simulink model "canTransceiverModel"  (R2018a)
settings: Solver=FixedStepDiscrete  StartTime=0.0  StopTime=50  RelTol=1e-3  EnableMultiTasking=on
values from neighbouring files (symbols this model uses):
  sampleTime = 0.040    (= 0.04)    [canTrasceiverConfig.m]
  sensorLocationConfig = uint8(sensorLocationConfig)    [canTrasceiverConfig.m]
undefined symbols (not defined in the file or in its folder): canChannel, CRC
libraries: simulink x81, canmsglib x27, canlib x8, commcrc2 x1
(part 1 of 5)
settings Model: FPTRunName=Active  Creator=The MathWorks, Inc.  LastModifiedBy=Giovanni
settings DataIOCC: LimitDataPoints=on  SaveFormat=Array
settings OptimizationCC: BlockReduction=off  ExpressionDepthLimit=2147483647  LifeSpan=inf
settings DebuggingCC: UnderspecifiedInitializationDetection=Classic  MergeDetectMultiDrivingBlocksExec=none  SolverPrmCheckMsg=warning  FcnCallInpInsideContextMsg=warning  StateNameClashWarn=warning  SFUnexpectedBacktrackingDiag=warning  SFNoUnconditionalDefaultTransitionDiag=warning  SFExecutionAtInitializationDiag=none
settings HardwareCC: ProdBitPerPointer=32  ProdBitPerSizeT=32  ProdBitPerPtrDiffT=32  ProdLargestAtomicFloat=None  ProdIntDivRoundTo=Undefined  ProdEndianess=Unspecified  ProdWordSize=32  ProdHWDeviceType=32-bit Generic
settings ModelReferenceCC: PropagateSignalLabelsOutOfModel=off
settings RTWCC: PostCodeGenCommand=packNGo(buildInfo)  Description=Generic Real-Time Target  RetainRTWFile=on  TLCDebug=on
settings CodeAppCC: StateflowObjectComments=on
settings GRTTargetCC: TargetLangStandard=C89/C90 (ANSI)  GeneratePreprocessorConditionals=Disable all  CombineOutputUpdateFcns=off  MatFileLogging=off  GRTInterface=on
settings ConfigComp: CovMetricSettings=dw  CovHtmlReporting=on  CovSaveCumulativeToWorkspaceVar=on  CovSaveSingleToWorkspaceVar=on  CovExternalEMLEnable=off

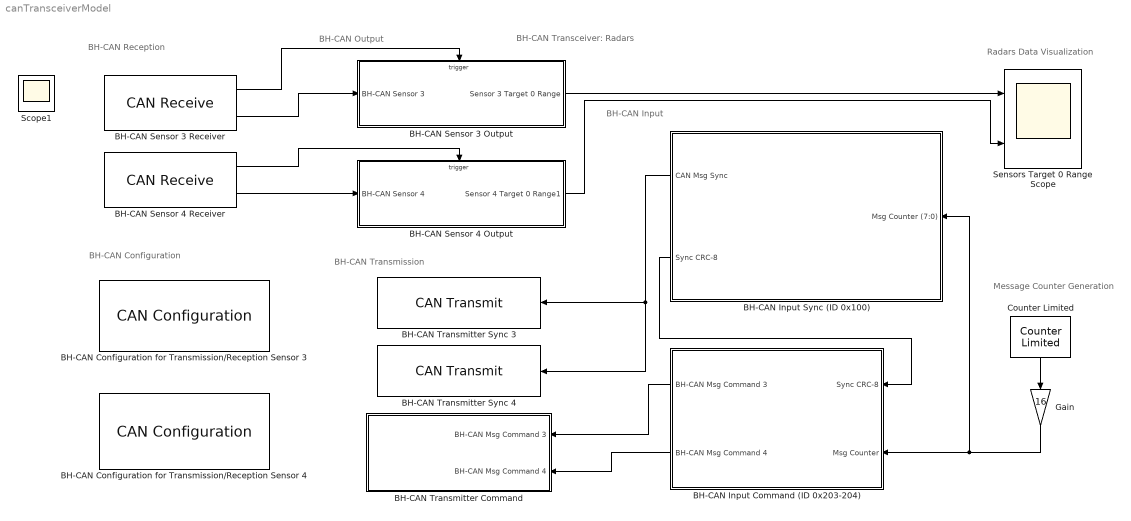
== system canTransceiverModel ==
  note: Radars Data Visualization
  note: BH-CAN Input
  note: BH-CAN Configuration
  note: BH-CAN Output
  note: BH-CAN Reception
  note: BH-CAN Transmission
  note: Message Counter
      | Generation
  note: BH-CAN Transceiver: Radars
  BH-CAN Configuration for Transmission/Reception Sensor 3 : canlib/CAN Configuration  BlockHandle=5.0001  DeviceMenu=MathWorks Virtual 1 (Channel 1)  Device=Vector VN1640A 1 (Channel 1)  ObjConstructor=canChannel('Vector','VN1640A 1',1)  BusSpeed=500000  EnableBitParameters=off  SJW=1  TSEG1=4  TSEG2=3  NSamples=1  AckMode=Normal
      settings: SourceProductName=Vehicle Network Toolbox  SourceProductBaseCode=VN
  BH-CAN Configuration for Transmission/Reception Sensor 4 : canlib/CAN Configuration  BlockHandle=6.0001  DeviceMenu=MathWorks Virtual 1 (Channel 1)  Device=Vector VN1640A 1 (Channel 2)  ObjConstructor=canChannel('Vector','VN1640A 1',2)  BusSpeed=500000  EnableBitParameters=off  SJW=1  TSEG1=4  TSEG2=3  NSamples=1  AckMode=Normal
      settings: SourceProductName=Vehicle Network Toolbox  SourceProductBaseCode=VN
  BH-CAN Input Command (ID 0x203-204) : Subsystem
  BH-CAN Input Sync (ID 0x100) : Subsystem
  BH-CAN Sensor 3 Output : Subsystem  TreatAsAtomicUnit=on
      settings: RTWSystemCode=Nonreusable function
  BH-CAN Sensor 3 Receiver : canlib/CAN Receive  BlockHandle=1800.0001  DeviceMenu=(none)  Device=Vector VN1640A 1 (Channel 1)  ObjConstructor=canChannel('Vector','VN1640A 1',1)  EnableStandardIDsFilter=off  StandardIDs=0  EnableExtendedIDsFilter=off  ExtendedIDs=0  SampleTime=sampleTime  MsgsPerTimestep=all  StdIDsCombo=Allow all  ExtIDsCombo=Allow all  InternalFilterUpdateStatus=on  BusOutput=off
      settings: SourceProductName=Vehicle Network Toolbox  SourceProductBaseCode=VN
  BH-CAN Sensor 4 Output : Subsystem  TreatAsAtomicUnit=on
      settings: RTWSystemCode=Nonreusable function
  BH-CAN Sensor 4 Receiver : canlib/CAN Receive  BlockHandle=3437.0001  DeviceMenu=MathWorks Virtual 1 (Channel 1)  Device=Vector VN1640A 1 (Channel 2)  ObjConstructor=canChannel('Vector','VN1640A 1',2)  EnableStandardIDsFilter=off  StandardIDs=0  EnableExtendedIDsFilter=off  ExtendedIDs=0  SampleTime=sampleTime  MsgsPerTimestep=all  StdIDsCombo=Allow all  ExtIDsCombo=Allow all  InternalFilterUpdateStatus=on  BusOutput=off
      settings: SourceProductName=Vehicle Network Toolbox  SourceProductBaseCode=VN
  BH-CAN Transmitter Command : Subsystem
  BH-CAN Transmitter Sync 3 : canlib/CAN Transmit  BlockHandle=3445.0001  DeviceMenu=MathWorks Virtual 1 (Channel 1)  Device=Vector VN1640A 1 (Channel 1)  ObjConstructor=canChannel('Vector','VN1640A 1',1)  EnablePeriodicTransmit=off  MessagePeriod=0.025
      settings: SourceProductName=Vehicle Network Toolbox  SourceProductBaseCode=VN
  BH-CAN Transmitter Sync 4 : canlib/CAN Transmit  BlockHandle=3446.0001  DeviceMenu=MathWorks Virtual 1 (Channel 1)  Device=Vector VN1640A 1 (Channel 2)  ObjConstructor=canChannel('Vector','VN1640A 1',2)  EnablePeriodicTransmit=off  MessagePeriod=0.025
      settings: SourceProductName=Vehicle Network Toolbox  SourceProductBaseCode=VN
  Counter Limited : simulink/Sources/Counter Limited  uplimit=15  tsamp=sampleTime
  Gain : Gain  Gain=16  OutDataTypeStr=Inherit: Same as input
  Sensors Target 0 Range Scope : Scope  NumInputPorts=2
  Scope1 : Scope
  wires:
  BH-CAN Input Sync (ID 0x100)/1(CAN Msg Sync) -> BH-CAN Transmitter Sync 3/1, BH-CAN Transmitter Sync 4/1
  Counter Limited/1 -> Gain/1
  Gain/1 -> BH-CAN Input Sync (ID 0x100)/1(Msg Counter (7:0)), BH-CAN Input Command (ID 0x203-204)/2(Msg Counter)
  BH-CAN Sensor 3 Receiver/2 -> BH-CAN Sensor 3 Output/1(BH-CAN Sensor 3)
  BH-CAN Sensor 3 Receiver/1 -> BH-CAN Sensor 3 Output/Trigger
  BH-CAN Sensor 4 Receiver/1 -> BH-CAN Sensor 4 Output/Trigger
  BH-CAN Sensor 4 Receiver/2 -> BH-CAN Sensor 4 Output/1(BH-CAN Sensor 4)
  BH-CAN Input Sync (ID 0x100)/2(Sync CRC-8) -> BH-CAN Input Command (ID 0x203-204)/1(Sync CRC-8)
  BH-CAN Input Command (ID 0x203-204)/1(BH-CAN Msg Command 3) -> BH-CAN Transmitter Command/1(BH-CAN Msg Command 3)
  BH-CAN Input Command (ID 0x203-204)/2(BH-CAN Msg Command 4) -> BH-CAN Transmitter Command/2(BH-CAN Msg Command 4)
  BH-CAN Sensor 3 Output/1(Sensor 3 Target 0 Range) -> Sensors Target 0 Range Scope/1
  BH-CAN Sensor 4 Output/1(Sensor 4 Target 0 Range1) -> Sensors Target 0 Range Scope/2

== system canTransceiverModel/BH-CAN Input Command (ID 0x203-204) ==
  Sync CRC-8 : Inport
  Msg Counter : Inport  Port=2
  BH-CAN Input Command 3 (ID 0x203) : Subsystem
  BH-CAN Input Command 4 (ID 0x204) : Subsystem
  BH-CAN Msg Command 3 : Outport
  BH-CAN Msg Command 4 : Outport  Port=2
  wires:
  Sync CRC-8/1 -> BH-CAN Input Command 4 (ID 0x204)/2(Sync Msg Content CRC-8 (7:0)), BH-CAN Input Command 3 (ID 0x203)/2(Sync Msg CRC-8 (7:0))
  BH-CAN Input Command 4 (ID 0x204)/1(CAN Msg Command 3) -> BH-CAN Msg Command 4/1
  BH-CAN Input Command 3 (ID 0x203)/1(CAN Msg Command 3) -> BH-CAN Msg Command 3/1
  Msg Counter/1 -> BH-CAN Input Command 3 (ID 0x203)/1(Msg Counter (7:0)), BH-CAN Input Command 4 (ID 0x204)/1(Msg Counter (7:0))

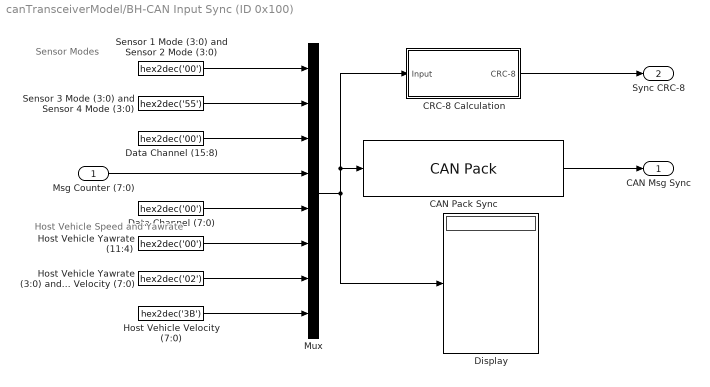
== system canTransceiverModel/BH-CAN Input Sync (ID 0x100) ==
  note: Host Vehicle
      | Speed and
      | Yawrate
  note: Sensor Modes
  Msg Counter (7:0) : Inport
  CAN Pack Sync : canmsglib/CAN Pack  MsgList=(none)  MsgName=CAN Msg  MsgIDType=Standard (11-bit identifier)  MsgIdentifier=hex2dec('100')  MsgLength=8  NSignals=0  StartBits=0  SignalSizes=0  ByteOrders=0  DataTypes=0  MultiplexTypes=0  MultiplexValues=0  Factors=0  Offsets=0  Minimums=0  Maximums=0  Remote=off  ApplyMinMax=off  BusOutput=off
      settings: SourceProductName=Simulink Real-Time  SourceProductBaseCode=XP  DataFormat=raw data
  CRC-8 Calculation : Subsystem
  Data Channel (15:8) : Constant  Value=hex2dec('00')  OutDataTypeStr=uint8  SampleTime=sampleTime
  Data Channel (7:0) : Constant  Value=hex2dec('00')  OutDataTypeStr=uint8  SampleTime=sampleTime
  Display : Display
  Host Vehicle Velocity (7:0) : Constant  Value=hex2dec('3B')  OutDataTypeStr=uint8  SampleTime=sampleTime
  Host Vehicle Yawrate (11:4) : Constant  Value=hex2dec('00')  OutDataTypeStr=uint8  SampleTime=sampleTime
  Host Vehicle Yawrate (3:0) and Velocity (7:0) : Constant  Value=hex2dec('02')  OutDataTypeStr=uint8  SampleTime=sampleTime
  Mux : Mux  Inputs=8
  Sensor 1 Mode (3:0) and Sensor 2 Mode (3:0) : Constant  Value=hex2dec('00')  OutDataTypeStr=uint8  SampleTime=sampleTime
  Sensor 3 Mode (3:0) and Sensor 4 Mode (3:0) : Constant  Value=hex2dec('55')  OutDataTypeStr=uint8  SampleTime=sampleTime
  CAN Msg Sync : Outport
  Sync CRC-8 : Outport  Port=2
  wires:
  CAN Pack Sync/1 -> CAN Msg Sync/1
  Mux/1 -> CRC-8 Calculation/1(Input), CAN Pack Sync/1, Display/1
  Sensor 1 Mode (3:0) and Sensor 2 Mode (3:0)/1 -> Mux/1
  Sensor 3 Mode (3:0) and Sensor 4 Mode (3:0)/1 -> Mux/2
  Data Channel (15:8)/1 -> Mux/3
  Data Channel (7:0)/1 -> Mux/5
  Host Vehicle Yawrate (11:4)/1 -> Mux/6
  Host Vehicle Yawrate (3:0) and Velocity (7:0)/1 -> Mux/7
  Host Vehicle Velocity (7:0)/1 -> Mux/8
  Msg Counter (7:0)/1 -> Mux/4
  CRC-8 Calculation/1(CRC-8) -> Sync CRC-8/1

== system canTransceiverModel/BH-CAN Sensor 3 Output ==
  BH-CAN Sensor 3 : Inport
  function : TriggerPort  TriggerType=function-call  VariantControl=Variant
  Command Sensor 3 (ID 0x203) : Subsystem  VariantControl=Variant1
  Sync (ID 0x100) : Subsystem
  Targets 0-9 (ID 0x300-309) : Subsystem
  Sensor 3 Target 0 Range : Outport
  wires:
  BH-CAN Sensor 3/1 -> Sync (ID 0x100)/1(CAN Msg), Command Sensor 3 (ID 0x203)/1(CAN Msg), Targets 0-9 (ID 0x300-309)/1(CAN Msg)
  Targets 0-9 (ID 0x300-309)/1(Sensor 3 Target 0 Range) -> Sensor 3 Target 0 Range/1

== system canTransceiverModel/BH-CAN Sensor 4 Output ==
  BH-CAN Sensor 4 : Inport
  function : TriggerPort  TriggerType=function-call  VariantControl=Variant
  Command Sensor 4 (ID 0x204) : Subsystem  VariantControl=Variant1
  Sync (ID 0x100) : Subsystem
  Targets 0-9 (ID 0x300-309) : Subsystem
  Sensor 4 Target 0 Range1 : Outport
  wires:
  BH-CAN Sensor 4/1 -> Sync (ID 0x100)/1(CAN Msg), Command Sensor 4 (ID 0x204)/1(CAN Msg), Targets 0-9 (ID 0x300-309)/1(CAN Msg)
  Targets 0-9 (ID 0x300-309)/1(Sensor 4 Target 0 Range1) -> Sensor 4 Target 0 Range1/1

== system canTransceiverModel/BH-CAN Transmitter Command ==
  BH-CAN Msg Command 3 : Inport
  BH-CAN Msg Command 4 : Inport  Port=2
  BH-CAN Transmitter Command 3 : canlib/CAN Transmit  BlockHandle=3441.0001  DeviceMenu=MathWorks Virtual 1 (Channel 1)  Device=Vector VN1640A 1 (Channel 1)  ObjConstructor=canChannel('Vector','VN1640A 1',1)  EnablePeriodicTransmit=off  MessagePeriod=0.025
      settings: SourceProductName=Vehicle Network Toolbox  SourceProductBaseCode=VN
  BH-CAN Transmitter Command 4 : canlib/CAN Transmit  BlockHandle=3442.0001  DeviceMenu=MathWorks Virtual 1 (Channel 1)  Device=Vector VN1640A 1 (Channel 2)  ObjConstructor=canChannel('Vector','VN1640A 1',2)  EnablePeriodicTransmit=off  MessagePeriod=0.025
      settings: SourceProductName=Vehicle Network Toolbox  SourceProductBaseCode=VN
  wires:
  BH-CAN Msg Command 3/1 -> BH-CAN Transmitter Command 3/1
  BH-CAN Msg Command 4/1 -> BH-CAN Transmitter Command 4/1

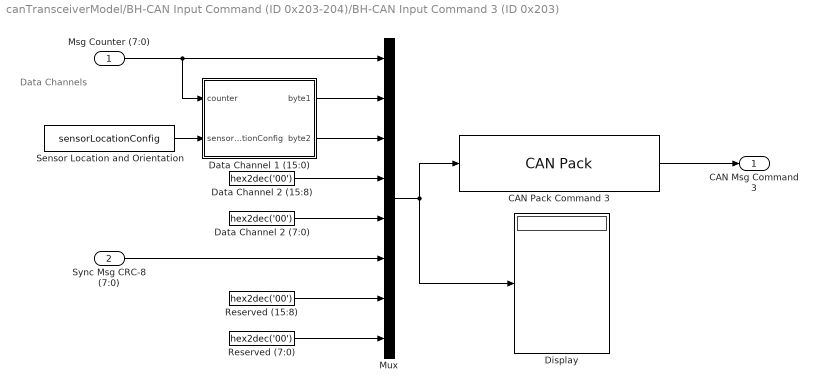
== system canTransceiverModel/BH-CAN Input Command (ID 0x203-204)/BH-CAN Input Command 3 (ID 0x203) ==
  note: Data Channels
  Msg Counter (7:0) : Inport
  Sync Msg CRC-8 (7:0) : Inport  Port=2
  CAN Pack Command 3 : canmsglib/CAN Pack  MsgList=(none)  MsgName=CAN Msg  MsgIDType=Standard (11-bit identifier)  MsgIdentifier=hex2dec('203')  MsgLength=8  NSignals=0  StartBits=0  SignalSizes=0  ByteOrders=0  DataTypes=0  MultiplexTypes=0  MultiplexValues=0  Factors=0  Offsets=0  Minimums=0  Maximums=0  Remote=off  ApplyMinMax=off  BusOutput=off
      settings: SourceProductName=Simulink Real-Time  SourceProductBaseCode=XP  DataFormat=raw data
  Data Channel 1 (15:0) : MATLAB Function  TreatAsAtomicUnit=on
  Data Channel 2 (15:8) : Constant  Value=hex2dec('00')  OutDataTypeStr=uint8  SampleTime=sampleTime
  Data Channel 2 (7:0) : Constant  Value=hex2dec('00')  OutDataTypeStr=uint8  SampleTime=sampleTime
  Display : Display
  Mux : Mux  Inputs=8
  Reserved (15:8) : Constant  Value=hex2dec('00')  OutDataTypeStr=uint8  SampleTime=sampleTime
  Reserved (7:0) : Constant  Value=hex2dec('00')  OutDataTypeStr=uint8  SampleTime=sampleTime
  Sensor Location and Orientation : Constant  Value=sensorLocationConfig  VectorParams1D=off  SampleTime=sampleTime
  CAN Msg Command 3 : Outport
  wires:
  CAN Pack Command 3/1 -> CAN Msg Command 3/1
  Data Channel 1 (15:0)/1(byte1) -> Mux/2
  Data Channel 1 (15:0)/2(byte2) -> Mux/3
  Data Channel 2 (15:8)/1 -> Mux/4
  Sync Msg CRC-8 (7:0)/1 -> Mux/6
  Reserved (15:8)/1 -> Mux/7
  Reserved (7:0)/1 -> Mux/8
  Data Channel 2 (7:0)/1 -> Mux/5
  Msg Counter (7:0)/1 -> Data Channel 1 (15:0)/1(counter), Mux/1
  Mux/1 -> CAN Pack Command 3/1, Display/1
  Sensor Location and Orientation/1 -> Data Channel 1 (15:0)/2(sensorLocationConfig)

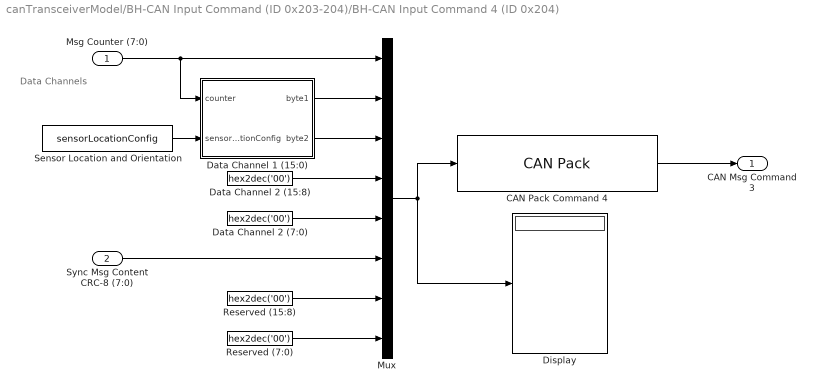
== system canTransceiverModel/BH-CAN Input Command (ID 0x203-204)/BH-CAN Input Command 4 (ID 0x204) ==
  note: Data Channels
  Msg Counter (7:0) : Inport
  Sync Msg Content CRC-8 (7:0) : Inport  Port=2
  CAN Pack Command 4 : canmsglib/CAN Pack  MsgList=(none)  MsgName=CAN Msg  MsgIDType=Standard (11-bit identifier)  MsgIdentifier=hex2dec('204')  MsgLength=8  NSignals=0  StartBits=0  SignalSizes=0  ByteOrders=0  DataTypes=0  MultiplexTypes=0  MultiplexValues=0  Factors=0  Offsets=0  Minimums=0  Maximums=0  Remote=off  ApplyMinMax=off  BusOutput=off
      settings: SourceProductName=Simulink Real-Time  SourceProductBaseCode=XP  DataFormat=raw data
  Data Channel 1 (15:0) : MATLAB Function  TreatAsAtomicUnit=on
  Data Channel 2 (15:8) : Constant  Value=hex2dec('00')  OutDataTypeStr=uint8  SampleTime=sampleTime
  Data Channel 2 (7:0) : Constant  Value=hex2dec('00')  OutDataTypeStr=uint8  SampleTime=sampleTime
  Display : Display
  Mux : Mux  Inputs=8
  Reserved (15:8) : Constant  Value=hex2dec('00')  OutDataTypeStr=uint8  SampleTime=sampleTime
  Reserved (7:0) : Constant  Value=hex2dec('00')  OutDataTypeStr=uint8  SampleTime=sampleTime
  Sensor Location and Orientation : Constant  Value=sensorLocationConfig  VectorParams1D=off  SampleTime=sampleTime
  CAN Msg Command 3 : Outport
  wires:
  CAN Pack Command 4/1 -> CAN Msg Command 3/1
  Data Channel 1 (15:0)/1(byte1) -> Mux/2
  Data Channel 1 (15:0)/2(byte2) -> Mux/3
  Data Channel 2 (15:8)/1 -> Mux/4
  Sync Msg Content CRC-8 (7:0)/1 -> Mux/6
  Reserved (15:8)/1 -> Mux/7
  Reserved (7:0)/1 -> Mux/8
  Data Channel 2 (7:0)/1 -> Mux/5
  Msg Counter (7:0)/1 -> Data Channel 1 (15:0)/1(counter), Mux/1
  Mux/1 -> CAN Pack Command 4/1, Display/1
  Sensor Location and Orientation/1 -> Data Channel 1 (15:0)/2(sensorLocationConfig)

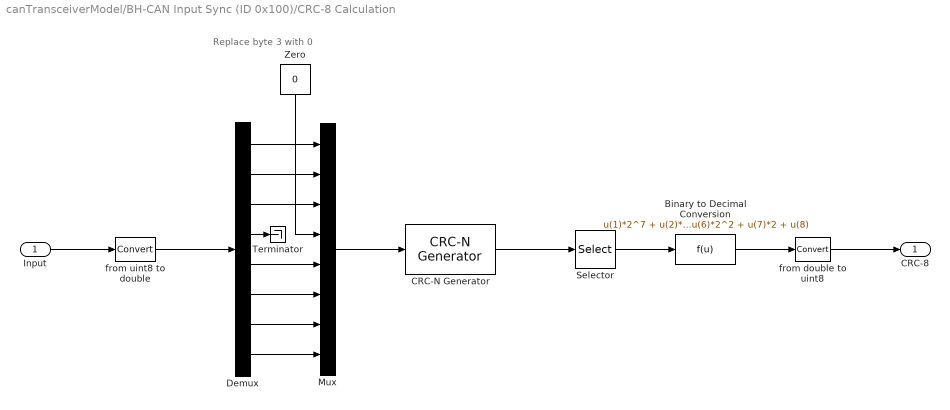
== system canTransceiverModel/BH-CAN Input Sync (ID 0x100)/CRC-8 Calculation ==
  note: Replace byte 3 with 0
  Input : Inport
  Binary to Decimal Conversion : Fcn  Expr=u(1)*2^7 + u(2)*2^6 + u(3)*2^5 + u(4)*2^4 + u(5)*2^3 + u(6)*2^2 + u(7)*2 + u(8)
  CRC-N Generator : commcrc2/CRC-N Generator  crcMethod=CRC-8  iniStates=[0]  numChecksums=1
      settings: SourceProductName=Communications System Toolbox  SourceProductBaseCode=CM
  Demux : Demux  Outputs=8
  Mux : Mux  Inputs=8
  Selector : Selector  InputPortWidth=16  IndexOptions=Index vector (dialog)  Indices=[9:16]  OutputSizes=1
  Terminator : Terminator
  Zero : Constant  Value=0  SampleTime=sampleTime
  from double to uint8 : DataTypeConversion
  from uint8 to double : DataTypeConversion
  CRC-8 : Outport
  wires:
  CRC-N Generator/1 -> Selector/1
  Binary to Decimal Conversion/1 -> from double to uint8/1
  Selector/1 -> Binary to Decimal Conversion/1
  from uint8 to double/1 -> Demux/1
  Input/1 -> from uint8 to double/1
  from double to uint8/1 -> CRC-8/1
  Mux/1 -> CRC-N Generator/1
  Demux/1 -> Mux/1
  Demux/2 -> Mux/2
  Demux/3 -> Mux/3
  Demux/5 -> Mux/5
  Demux/6 -> Mux/6
  Demux/7 -> Mux/7
  Demux/8 -> Mux/8
  Demux/4 -> Terminator/1
  Zero/1 -> Mux/4

== system canTransceiverModel/BH-CAN Sensor 3 Output/Command Sensor 3 (ID 0x203) ==
  CAN Msg : Inport
  CAN Unpack Command 3 : canmsglib/CAN Unpack  CANdbFile=VehicleInfo.dbc  MsgList=WheelSpeeds  MsgName=Command 3  MsgIDType=Standard (11-bit identifier)  MsgIdentifier=hex2dec('203')  MsgLength=8  SignalInfo=LF_WSpeed$8$16$2$2$1$0$1.000000e-02$-100$0$2000$#LR_WSpeed$40$16$2$2$1$0$1.000000e-02$-100$0$2000$#RF_WSpeed$24$16$2$2$1$0$1.000000e-02$-100$0$2000$#RR_WSpeed$56$16$2$2$1$0$1.000000e-02$-100$0$2000$#  NSignals=4  IDPort=off  TimestampPort=off  ErrorPort=off  RemotePort=off  LengthPort=off  StatusPort=off  StartBits=str2num('[int32(8);int32(40);int32(24);int32(56)]')  SignalSizes=str2num('[int32(16);int32(16);int32(16);int32(16)]')  ByteOrders=str2num('[int32(2);int32(2);int32(2);int32(2)]')  DataTypes=str2num('[int32(2);int32(2);int32(2);int32(2)]')  MultiplexTypes=str2num('[int32(1);int32(1);int32(1);int32(1)]')  MultiplexValues=str2num('[double(0);double(0);double(0);double(0)]')  Factors=str2num('[double(1.000000e-02);double(1.000000e-02);double(1.000000e-02);double(1.000000e-02)]')  Offsets=str2num('[double(-100);double(-100);double(-100);double(-100)]')  Minimums=str2num('[double(0);double(0);double(0);double(0)]')  Maximums=str2num('[double(2000);double(2000);double(2000);double(2000)]')  ApplyMinMax=off
      settings: SourceProductName=Simulink Real-Time  SourceProductBaseCode=XP  DataFormat=raw data
  Display Command 3 : Display
      settings: Format=hex (Stored Integer)
  wires:
  CAN Unpack Command 3/1 -> Display Command 3/1
  CAN Msg/1 -> CAN Unpack Command 3/1

== system canTransceiverModel/BH-CAN Sensor 3 Output/Sync (ID 0x100) ==
  CAN Msg : Inport
  CAN Unpack Sync : canmsglib/CAN Unpack  CANdbFile=VehicleInfo.dbc  MsgList=WheelSpeeds  MsgName=Sync  MsgIDType=Standard (11-bit identifier)  MsgIdentifier=hex2dec('100')  MsgLength=8  SignalInfo=LF_WSpeed$8$16$2$2$1$0$1.000000e-02$-100$0$2000$#LR_WSpeed$40$16$2$2$1$0$1.000000e-02$-100$0$2000$#RF_WSpeed$24$16$2$2$1$0$1.000000e-02$-100$0$2000$#RR_WSpeed$56$16$2$2$1$0$1.000000e-02$-100$0$2000$#  NSignals=4  IDPort=off  TimestampPort=off  ErrorPort=off  RemotePort=off  LengthPort=off  StatusPort=off  StartBits=str2num('[int32(8);int32(40);int32(24);int32(56)]')  SignalSizes=str2num('[int32(16);int32(16);int32(16);int32(16)]')  ByteOrders=str2num('[int32(2);int32(2);int32(2);int32(2)]')  DataTypes=str2num('[int32(2);int32(2);int32(2);int32(2)]')  MultiplexTypes=str2num('[int32(1);int32(1);int32(1);int32(1)]')  MultiplexValues=str2num('[double(0);double(0);double(0);double(0)]')  Factors=str2num('[double(1.000000e-02);double(1.000000e-02);double(1.000000e-02);double(1.000000e-02)]')  Offsets=str2num('[double(-100);double(-100);double(-100);double(-100)]')  Minimums=str2num('[double(0);double(0);double(0);double(0)]')  Maximums=str2num('[double(2000);double(2000);double(2000);double(2000)]')  ApplyMinMax=off
      settings: SourceProductName=Simulink Real-Time  SourceProductBaseCode=XP  DataFormat=raw data
  Display Sync : Display
      settings: Format=hex (Stored Integer)
  wires:
  CAN Unpack Sync/1 -> Display Sync/1
  CAN Msg/1 -> CAN Unpack Sync/1

== system canTransceiverModel/BH-CAN Sensor 3 Output/Targets 0-9 (ID 0x300-309) ==
  note: Sensor 3 Raw Data
  CAN Msg : Inport
  CAN Unpack Targets : Subsystem
  Display Targets : Display
      settings: Format=hex (Stored Integer)
  Mux : Mux  Inputs=10
  Targets Range and Bearing Information : Subsystem
  Sensor 3 Target 0 Range : Outport
  wires:
  CAN Msg/1 -> CAN Unpack Targets/1(In1)
  Mux/1 -> Display Targets/1
  CAN Unpack Targets/3(Target 2) -> Targets Range and Bearing Information/3(CAN Target 2), Mux/3
  CAN Unpack Targets/4(Target 3) -> Mux/4, Targets Range and Bearing Information/4(CAN Target 3)
  CAN Unpack Targets/5(Target 4) -> Targets Range and Bearing Information/5(CAN Target 4), Mux/5
  CAN Unpack Targets/6(Target 5) -> Targets Range and Bearing Information/6(CAN Target 5), Mux/6
  CAN Unpack Targets/7(Target 6) -> Targets Range and Bearing Information/7(CAN Target 6), Mux/7
  CAN Unpack Targets/8(Target 7) -> Targets Range and Bearing Information/8(CAN Target 7), Mux/8
  CAN Unpack Targets/9(Target 8) -> Targets Range and Bearing Information/9(CAN Target 8), Mux/9
  CAN Unpack Targets/10(Target 9) -> Targets Range and Bearing Information/10(CAN Target 9), Mux/10
  CAN Unpack Targets/1(Target 0) -> Mux/1, Targets Range and Bearing Information/1(CAN Target 0)
  CAN Unpack Targets/2(Target 1) -> Mux/2, Targets Range and Bearing Information/2(CAN Target 1)
  Targets Range and Bearing Information/1(Sensor 3 Target 0 Range) -> Sensor 3 Target 0 Range/1

== system canTransceiverModel/BH-CAN Sensor 4 Output/Command Sensor 4 (ID 0x204) ==
  CAN Msg : Inport
  CAN Unpack Command 4 : canmsglib/CAN Unpack  CANdbFile=VehicleInfo.dbc  MsgList=WheelSpeeds  MsgName=Command 4  MsgIDType=Standard (11-bit identifier)  MsgIdentifier=hex2dec('204')  MsgLength=8  SignalInfo=LF_WSpeed$8$16$2$2$1$0$1.000000e-02$-100$0$2000$#LR_WSpeed$40$16$2$2$1$0$1.000000e-02$-100$0$2000$#RF_WSpeed$24$16$2$2$1$0$1.000000e-02$-100$0$2000$#RR_WSpeed$56$16$2$2$1$0$1.000000e-02$-100$0$2000$#  NSignals=4  IDPort=off  TimestampPort=off  ErrorPort=off  RemotePort=off  LengthPort=off  StatusPort=off  StartBits=str2num('[int32(8);int32(40);int32(24);int32(56)]')  SignalSizes=str2num('[int32(16);int32(16);int32(16);int32(16)]')  ByteOrders=str2num('[int32(2);int32(2);int32(2);int32(2)]')  DataTypes=str2num('[int32(2);int32(2);int32(2);int32(2)]')  MultiplexTypes=str2num('[int32(1);int32(1);int32(1);int32(1)]')  MultiplexValues=str2num('[double(0);double(0);double(0);double(0)]')  Factors=str2num('[double(1.000000e-02);double(1.000000e-02);double(1.000000e-02);double(1.000000e-02)]')  Offsets=str2num('[double(-100);double(-100);double(-100);double(-100)]')  Minimums=str2num('[double(0);double(0);double(0);double(0)]')  Maximums=str2num('[double(2000);double(2000);double(2000);double(2000)]')  ApplyMinMax=off
      settings: SourceProductName=Simulink Real-Time  SourceProductBaseCode=XP  DataFormat=raw data
  Display Command 4 : Display
      settings: Format=hex (Stored Integer)
  wires:
  CAN Unpack Command 4/1 -> Display Command 4/1
  CAN Msg/1 -> CAN Unpack Command 4/1

== system canTransceiverModel/BH-CAN Sensor 4 Output/Sync (ID 0x100) ==
  CAN Msg : Inport
  CAN Unpack Sync : canmsglib/CAN Unpack  CANdbFile=VehicleInfo.dbc  MsgList=WheelSpeeds  MsgName=Sync  MsgIDType=Standard (11-bit identifier)  MsgIdentifier=hex2dec('100')  MsgLength=8  SignalInfo=LF_WSpeed$8$16$2$2$1$0$1.000000e-02$-100$0$2000$#LR_WSpeed$40$16$2$2$1$0$1.000000e-02$-100$0$2000$#RF_WSpeed$24$16$2$2$1$0$1.000000e-02$-100$0$2000$#RR_WSpeed$56$16$2$2$1$0$1.000000e-02$-100$0$2000$#  NSignals=4  IDPort=off  TimestampPort=off  ErrorPort=off  RemotePort=off  LengthPort=off  StatusPort=off  StartBits=str2num('[int32(8);int32(40);int32(24);int32(56)]')  SignalSizes=str2num('[int32(16);int32(16);int32(16);int32(16)]')  ByteOrders=str2num('[int32(2);int32(2);int32(2);int32(2)]')  DataTypes=str2num('[int32(2);int32(2);int32(2);int32(2)]')  MultiplexTypes=str2num('[int32(1);int32(1);int32(1);int32(1)]')  MultiplexValues=str2num('[double(0);double(0);double(0);double(0)]')  Factors=str2num('[double(1.000000e-02);double(1.000000e-02);double(1.000000e-02);double(1.000000e-02)]')  Offsets=str2num('[double(-100);double(-100);double(-100);double(-100)]')  Minimums=str2num('[double(0);double(0);double(0);double(0)]')  Maximums=str2num('[double(2000);double(2000);double(2000);double(2000)]')  ApplyMinMax=off
      settings: SourceProductName=Simulink Real-Time  SourceProductBaseCode=XP  DataFormat=raw data
  Display Sync : Display
      settings: Format=hex (Stored Integer)
  wires:
  CAN Unpack Sync/1 -> Display Sync/1
  CAN Msg/1 -> CAN Unpack Sync/1

== system canTransceiverModel/BH-CAN Sensor 4 Output/Targets 0-9 (ID 0x300-309) ==
  note: Sensor 4 Raw Data
  CAN Msg : Inport
  CAN Unpack Targets : Subsystem
  Display Targets : Display
      settings: Format=hex (Stored Integer)
  Mux : Mux  Inputs=10
  Targets Range and Bearing Information : Subsystem
  Sensor 4 Target 0 Range1 : Outport
  wires:
  CAN Msg/1 -> CAN Unpack Targets/1(In1)
  Mux/1 -> Display Targets/1
  CAN Unpack Targets/3(Target 2) -> Targets Range and Bearing Information/3(CAN Target 2), Mux/3
  CAN Unpack Targets/4(Target 3) -> Mux/4, Targets Range and Bearing Information/4(CAN Target 3)
  CAN Unpack Targets/5(Target 4) -> Targets Range and Bearing Information/5(CAN Target 4), Mux/5
  CAN Unpack Targets/6(Target 5) -> Targets Range and Bearing Information/6(CAN Target 5), Mux/6
  CAN Unpack Targets/7(Target 6) -> Targets Range and Bearing Information/7(CAN Target 6), Mux/7
  CAN Unpack Targets/8(Target 7) -> Targets Range and Bearing Information/8(CAN Target 7), Mux/8
  CAN Unpack Targets/9(Target 8) -> Targets Range and Bearing Information/9(CAN Target 8), Mux/9
  CAN Unpack Targets/10(Target 9) -> Targets Range and Bearing Information/10(CAN Target 9), Mux/10
  CAN Unpack Targets/1(Target 0) -> Mux/1, Targets Range and Bearing Information/1(CAN Target 0)
  CAN Unpack Targets/2(Target 1) -> Mux/2, Targets Range and Bearing Information/2(CAN Target 1)
  Targets Range and Bearing Information/1(Sensor 4 Target 0 Range) -> Sensor 4 Target 0 Range1/1

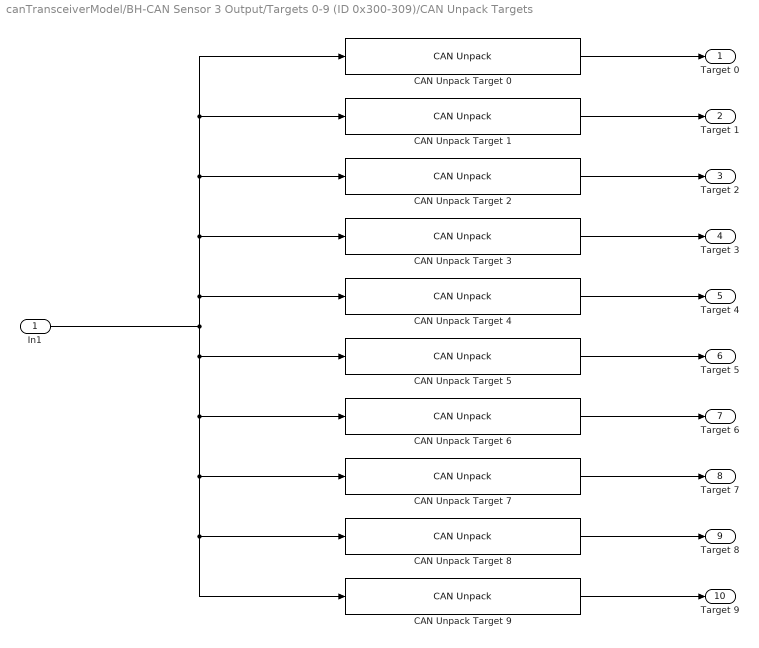
== system canTransceiverModel/BH-CAN Sensor 3 Output/Targets 0-9 (ID 0x300-309)/CAN Unpack Targets ==
  In1 : Inport
  CAN Unpack Target 0 : canmsglib/CAN Unpack  CANdbFile=VehicleInfo.dbc  MsgList=WheelSpeeds  MsgName=Target 0  MsgIDType=Standard (11-bit identifier)  MsgIdentifier=hex2dec('300')  MsgLength=8  SignalInfo=LF_WSpeed$8$16$2$2$1$0$1.000000e-02$-100$0$2000$#LR_WSpeed$40$16$2$2$1$0$1.000000e-02$-100$0$2000$#RF_WSpeed$24$16$2$2$1$0$1.000000e-02$-100$0$2000$#RR_WSpeed$56$16$2$2$1$0$1.000000e-02$-100$0$2000$#  NSignals=4  IDPort=off  TimestampPort=off  ErrorPort=off  RemotePort=off  LengthPort=off  StatusPort=off  StartBits=str2num('[int32(8);int32(40);int32(24);int32(56)]')  SignalSizes=str2num('[int32(16);int32(16);int32(16);int32(16)]')  ByteOrders=str2num('[int32(2);int32(2);int32(2);int32(2)]')  DataTypes=str2num('[int32(2);int32(2);int32(2);int32(2)]')  MultiplexTypes=str2num('[int32(1);int32(1);int32(1);int32(1)]')  MultiplexValues=str2num('[double(0);double(0);double(0);double(0)]')  Factors=str2num('[double(1.000000e-02);double(1.000000e-02);double(1.000000e-02);double(1.000000e-02)]')  Offsets=str2num('[double(-100);double(-100);double(-100);double(-100)]')  Minimums=str2num('[double(0);double(0);double(0);double(0)]')  Maximums=str2num('[double(2000);double(2000);double(2000);double(2000)]')  ApplyMinMax=off
      settings: SourceProductName=Simulink Real-Time  SourceProductBaseCode=XP  DataFormat=raw data
  CAN Unpack Target 1 : canmsglib/CAN Unpack  CANdbFile=VehicleInfo.dbc  MsgList=WheelSpeeds  MsgName=Target 1  MsgIDType=Standard (11-bit identifier)  MsgIdentifier=hex2dec('301')  MsgLength=8  SignalInfo=LF_WSpeed$8$16$2$2$1$0$1.000000e-02$-100$0$2000$#LR_WSpeed$40$16$2$2$1$0$1.000000e-02$-100$0$2000$#RF_WSpeed$24$16$2$2$1$0$1.000000e-02$-100$0$2000$#RR_WSpeed$56$16$2$2$1$0$1.000000e-02$-100$0$2000$#  NSignals=4  IDPort=off  TimestampPort=off  ErrorPort=off  RemotePort=off  LengthPort=off  StatusPort=off  StartBits=str2num('[int32(8);int32(40);int32(24);int32(56)]')  SignalSizes=str2num('[int32(16);int32(16);int32(16);int32(16)]')  ByteOrders=str2num('[int32(2);int32(2);int32(2);int32(2)]')  DataTypes=str2num('[int32(2);int32(2);int32(2);int32(2)]')  MultiplexTypes=str2num('[int32(1);int32(1);int32(1);int32(1)]')  MultiplexValues=str2num('[double(0);double(0);double(0);double(0)]')  Factors=str2num('[double(1.000000e-02);double(1.000000e-02);double(1.000000e-02);double(1.000000e-02)]')  Offsets=str2num('[double(-100);double(-100);double(-100);double(-100)]')  Minimums=str2num('[double(0);double(0);double(0);double(0)]')  Maximums=str2num('[double(2000);double(2000);double(2000);double(2000)]')  ApplyMinMax=off
      settings: SourceProductName=Simulink Real-Time  SourceProductBaseCode=XP  DataFormat=raw data
  CAN Unpack Target 2 : canmsglib/CAN Unpack  CANdbFile=VehicleInfo.dbc  MsgList=WheelSpeeds  MsgName=Target 2  MsgIDType=Standard (11-bit identifier)  MsgIdentifier=hex2dec('302')  MsgLength=8  SignalInfo=LF_WSpeed$8$16$2$2$1$0$1.000000e-02$-100$0$2000$#LR_WSpeed$40$16$2$2$1$0$1.000000e-02$-100$0$2000$#RF_WSpeed$24$16$2$2$1$0$1.000000e-02$-100$0$2000$#RR_WSpeed$56$16$2$2$1$0$1.000000e-02$-100$0$2000$#  NSignals=4  IDPort=off  TimestampPort=off  ErrorPort=off  RemotePort=off  LengthPort=off  StatusPort=off  StartBits=str2num('[int32(8);int32(40);int32(24);int32(56)]')  SignalSizes=str2num('[int32(16);int32(16);int32(16);int32(16)]')  ByteOrders=str2num('[int32(2);int32(2);int32(2);int32(2)]')  DataTypes=str2num('[int32(2);int32(2);int32(2);int32(2)]')  MultiplexTypes=str2num('[int32(1);int32(1);int32(1);int32(1)]')  MultiplexValues=str2num('[double(0);double(0);double(0);double(0)]')  Factors=str2num('[double(1.000000e-02);double(1.000000e-02);double(1.000000e-02);double(1.000000e-02)]')  Offsets=str2num('[double(-100);double(-100);double(-100);double(-100)]')  Minimums=str2num('[double(0);double(0);double(0);double(0)]')  Maximums=str2num('[double(2000);double(2000);double(2000);double(2000)]')  ApplyMinMax=off
      settings: SourceProductName=Simulink Real-Time  SourceProductBaseCode=XP  DataFormat=raw data
  CAN Unpack Target 3 : canmsglib/CAN Unpack  CANdbFile=VehicleInfo.dbc  MsgList=WheelSpeeds  MsgName=Target 3  MsgIDType=Standard (11-bit identifier)  MsgIdentifier=hex2dec('303')  MsgLength=8  SignalInfo=LF_WSpeed$8$16$2$2$1$0$1.000000e-02$-100$0$2000$#LR_WSpeed$40$16$2$2$1$0$1.000000e-02$-100$0$2000$#RF_WSpeed$24$16$2$2$1$0$1.000000e-02$-100$0$2000$#RR_WSpeed$56$16$2$2$1$0$1.000000e-02$-100$0$2000$#  NSignals=4  IDPort=off  TimestampPort=off  ErrorPort=off  RemotePort=off  LengthPort=off  StatusPort=off  StartBits=str2num('[int32(8);int32(40);int32(24);int32(56)]')  SignalSizes=str2num('[int32(16);int32(16);int32(16);int32(16)]')  ByteOrders=str2num('[int32(2);int32(2);int32(2);int32(2)]')  DataTypes=str2num('[int32(2);int32(2);int32(2);int32(2)]')  MultiplexTypes=str2num('[int32(1);int32(1);int32(1);int32(1)]')  MultiplexValues=str2num('[double(0);double(0);double(0);double(0)]')  Factors=str2num('[double(1.000000e-02);double(1.000000e-02);double(1.000000e-02);double(1.000000e-02)]')  Offsets=str2num('[double(-100);double(-100);double(-100);double(-100)]')  Minimums=str2num('[double(0);double(0);double(0);double(0)]')  Maximums=str2num('[double(2000);double(2000);double(2000);double(2000)]')  ApplyMinMax=off
      settings: SourceProductName=Simulink Real-Time  SourceProductBaseCode=XP  DataFormat=raw data
  CAN Unpack Target 4 : canmsglib/CAN Unpack  CANdbFile=VehicleInfo.dbc  MsgList=WheelSpeeds  MsgName=Target 4  MsgIDType=Standard (11-bit identifier)  MsgIdentifier=hex2dec('304')  MsgLength=8  SignalInfo=LF_WSpeed$8$16$2$2$1$0$1.000000e-02$-100$0$2000$#LR_WSpeed$40$16$2$2$1$0$1.000000e-02$-100$0$2000$#RF_WSpeed$24$16$2$2$1$0$1.000000e-02$-100$0$2000$#RR_WSpeed$56$16$2$2$1$0$1.000000e-02$-100$0$2000$#  NSignals=4  IDPort=off  TimestampPort=off  ErrorPort=off  RemotePort=off  LengthPort=off  StatusPort=off  StartBits=str2num('[int32(8);int32(40);int32(24);int32(56)]')  SignalSizes=str2num('[int32(16);int32(16);int32(16);int32(16)]')  ByteOrders=str2num('[int32(2);int32(2);int32(2);int32(2)]')  DataTypes=str2num('[int32(2);int32(2);int32(2);int32(2)]')  MultiplexTypes=str2num('[int32(1);int32(1);int32(1);int32(1)]')  MultiplexValues=str2num('[double(0);double(0);double(0);double(0)]')  Factors=str2num('[double(1.000000e-02);double(1.000000e-02);double(1.000000e-02);double(1.000000e-02)]')  Offsets=str2num('[double(-100);double(-100);double(-100);double(-100)]')  Minimums=str2num('[double(0);double(0);double(0);double(0)]')  Maximums=str2num('[double(2000);double(2000);double(2000);double(2000)]')  ApplyMinMax=off
      settings: SourceProductName=Simulink Real-Time  SourceProductBaseCode=XP  DataFormat=raw data
  CAN Unpack Target 5 : canmsglib/CAN Unpack  CANdbFile=VehicleInfo.dbc  MsgList=WheelSpeeds  MsgName=Target 5  MsgIDType=Standard (11-bit identifier)  MsgIdentifier=hex2dec('305')  MsgLength=8  SignalInfo=LF_WSpeed$8$16$2$2$1$0$1.000000e-02$-100$0$2000$#LR_WSpeed$40$16$2$2$1$0$1.000000e-02$-100$0$2000$#RF_WSpeed$24$16$2$2$1$0$1.000000e-02$-100$0$2000$#RR_WSpeed$56$16$2$2$1$0$1.000000e-02$-100$0$2000$#  NSignals=4  IDPort=off  TimestampPort=off  ErrorPort=off  RemotePort=off  LengthPort=off  StatusPort=off  StartBits=str2num('[int32(8);int32(40);int32(24);int32(56)]')  SignalSizes=str2num('[int32(16);int32(16);int32(16);int32(16)]')  ByteOrders=str2num('[int32(2);int32(2);int32(2);int32(2)]')  DataTypes=str2num('[int32(2);int32(2);int32(2);int32(2)]')  MultiplexTypes=str2num('[int32(1);int32(1);int32(1);int32(1)]')  MultiplexValues=str2num('[double(0);double(0);double(0);double(0)]')  Factors=str2num('[double(1.000000e-02);double(1.000000e-02);double(1.000000e-02);double(1.000000e-02)]')  Offsets=str2num('[double(-100);double(-100);double(-100);double(-100)]')  Minimums=str2num('[double(0);double(0);double(0);double(0)]')  Maximums=str2num('[double(2000);double(2000);double(2000);double(2000)]')  ApplyMinMax=off
      settings: SourceProductName=Simulink Real-Time  SourceProductBaseCode=XP  DataFormat=raw data
  CAN Unpack Target 6 : canmsglib/CAN Unpack  CANdbFile=VehicleInfo.dbc  MsgList=WheelSpeeds  MsgName=Target 6  MsgIDType=Standard (11-bit identifier)  MsgIdentifier=hex2dec('306')  MsgLength=8  SignalInfo=LF_WSpeed$8$16$2$2$1$0$1.000000e-02$-100$0$2000$#LR_WSpeed$40$16$2$2$1$0$1.000000e-02$-100$0$2000$#RF_WSpeed$24$16$2$2$1$0$1.000000e-02$-100$0$2000$#RR_WSpeed$56$16$2$2$1$0$1.000000e-02$-100$0$2000$#  NSignals=4  IDPort=off  TimestampPort=off  ErrorPort=off  RemotePort=off  LengthPort=off  StatusPort=off  StartBits=str2num('[int32(8);int32(40);int32(24);int32(56)]')  SignalSizes=str2num('[int32(16);int32(16);int32(16);int32(16)]')  ByteOrders=str2num('[int32(2);int32(2);int32(2);int32(2)]')  DataTypes=str2num('[int32(2);int32(2);int32(2);int32(2)]')  MultiplexTypes=str2num('[int32(1);int32(1);int32(1);int32(1)]')  MultiplexValues=str2num('[double(0);double(0);double(0);double(0)]')  Factors=str2num('[double(1.000000e-02);double(1.000000e-02);double(1.000000e-02);double(1.000000e-02)]')  Offsets=str2num('[double(-100);double(-100);double(-100);double(-100)]')  Minimums=str2num('[double(0);double(0);double(0);double(0)]')  Maximums=str2num('[double(2000);double(2000);double(2000);double(2000)]')  ApplyMinMax=off
      settings: SourceProductName=Simulink Real-Time  SourceProductBaseCode=XP  DataFormat=raw data
  CAN Unpack Target 7 : canmsglib/CAN Unpack  CANdbFile=VehicleInfo.dbc  MsgList=WheelSpeeds  MsgName=Target 7  MsgIDType=Standard (11-bit identifier)  MsgIdentifier=hex2dec('307')  MsgLength=8  SignalInfo=LF_WSpeed$8$16$2$2$1$0$1.000000e-02$-100$0$2000$#LR_WSpeed$40$16$2$2$1$0$1.000000e-02$-100$0$2000$#RF_WSpeed$24$16$2$2$1$0$1.000000e-02$-100$0$2000$#RR_WSpeed$56$16$2$2$1$0$1.000000e-02$-100$0$2000$#  NSignals=4  IDPort=off  TimestampPort=off  ErrorPort=off  RemotePort=off  LengthPort=off  StatusPort=off  StartBits=str2num('[int32(8);int32(40);int32(24);int32(56)]')  SignalSizes=str2num('[int32(16);int32(16);int32(16);int32(16)]')  ByteOrders=str2num('[int32(2);int32(2);int32(2);int32(2)]')  DataTypes=str2num('[int32(2);int32(2);int32(2);int32(2)]')  MultiplexTypes=str2num('[int32(1);int32(1);int32(1);int32(1)]')  MultiplexValues=str2num('[double(0);double(0);double(0);double(0)]')  Factors=str2num('[double(1.000000e-02);double(1.000000e-02);double(1.000000e-02);double(1.000000e-02)]')  Offsets=str2num('[double(-100);double(-100);double(-100);double(-100)]')  Minimums=str2num('[double(0);double(0);double(0);double(0)]')  Maximums=str2num('[double(2000);double(2000);double(2000);double(2000)]')  ApplyMinMax=off
      settings: SourceProductName=Simulink Real-Time  SourceProductBaseCode=XP  DataFormat=raw data
  CAN Unpack Target 8 : canmsglib/CAN Unpack  CANdbFile=VehicleInfo.dbc  MsgList=WheelSpeeds  MsgName=Target 8  MsgIDType=Standard (11-bit identifier)  MsgIdentifier=hex2dec('308')  MsgLength=8  SignalInfo=LF_WSpeed$8$16$2$2$1$0$1.000000e-02$-100$0$2000$#LR_WSpeed$40$16$2$2$1$0$1.000000e-02$-100$0$2000$#RF_WSpeed$24$16$2$2$1$0$1.000000e-02$-100$0$2000$#RR_WSpeed$56$16$2$2$1$0$1.000000e-02$-100$0$2000$#  NSignals=4  IDPort=off  TimestampPort=off  ErrorPort=off  RemotePort=off  LengthPort=off  StatusPort=off  StartBits=str2num('[int32(8);int32(40);int32(24);int32(56)]')  SignalSizes=str2num('[int32(16);int32(16);int32(16);int32(16)]')  ByteOrders=str2num('[int32(2);int32(2);int32(2);int32(2)]')  DataTypes=str2num('[int32(2);int32(2);int32(2);int32(2)]')  MultiplexTypes=str2num('[int32(1);int32(1);int32(1);int32(1)]')  MultiplexValues=str2num('[double(0);double(0);double(0);double(0)]')  Factors=str2num('[double(1.000000e-02);double(1.000000e-02);double(1.000000e-02);double(1.000000e-02)]')  Offsets=str2num('[double(-100);double(-100);double(-100);double(-100)]')  Minimums=str2num('[double(0);double(0);double(0);double(0)]')  Maximums=str2num('[double(2000);double(2000);double(2000);double(2000)]')  ApplyMinMax=off
      settings: SourceProductName=Simulink Real-Time  SourceProductBaseCode=XP  DataFormat=raw data
  CAN Unpack Target 9 : canmsglib/CAN Unpack  CANdbFile=VehicleInfo.dbc  MsgList=WheelSpeeds  MsgName=Target 9  MsgIDType=Standard (11-bit identifier)  MsgIdentifier=hex2dec('309')  MsgLength=8  SignalInfo=LF_WSpeed$8$16$2$2$1$0$1.000000e-02$-100$0$2000$#LR_WSpeed$40$16$2$2$1$0$1.000000e-02$-100$0$2000$#RF_WSpeed$24$16$2$2$1$0$1.000000e-02$-100$0$2000$#RR_WSpeed$56$16$2$2$1$0$1.000000e-02$-100$0$2000$#  NSignals=4  IDPort=off  TimestampPort=off  ErrorPort=off  RemotePort=off  LengthPort=off  StatusPort=off  StartBits=str2num('[int32(8);int32(40);int32(24);int32(56)]')  SignalSizes=str2num('[int32(16);int32(16);int32(16);int32(16)]')  ByteOrders=str2num('[int32(2);int32(2);int32(2);int32(2)]')  DataTypes=str2num('[int32(2);int32(2);int32(2);int32(2)]')  MultiplexTypes=str2num('[int32(1);int32(1);int32(1);int32(1)]')  MultiplexValues=str2num('[double(0);double(0);double(0);double(0)]')  Factors=str2num('[double(1.000000e-02);double(1.000000e-02);double(1.000000e-02);double(1.000000e-02)]')  Offsets=str2num('[double(-100);double(-100);double(-100);double(-100)]')  Minimums=str2num('[double(0);double(0);double(0);double(0)]')  Maximums=str2num('[double(2000);double(2000);double(2000);double(2000)]')  ApplyMinMax=off
      settings: SourceProductName=Simulink Real-Time  SourceProductBaseCode=XP  DataFormat=raw data
  Target 0 : Outport
  Target 1 : Outport  Port=2
  Target 2 : Outport  Port=3
  Target 3 : Outport  Port=4
  Target 4 : Outport  Port=5
  Target 5 : Outport  Port=6
  Target 6 : Outport  Port=7
  Target 7 : Outport  Port=8
  Target 8 : Outport  Port=9
  Target 9 : Outport  Port=10
  wires:
  In1/1 -> CAN Unpack Target 0/1, CAN Unpack Target 1/1, CAN Unpack Target 2/1, CAN Unpack Target 3/1, CAN Unpack Target 4/1, CAN Unpack Target 9/1, CAN Unpack Target 8/1, CAN Unpack Target 7/1, CAN Unpack Target 6/1, CAN Unpack Target 5/1
  CAN Unpack Target 3/1 -> Target 3/1
  CAN Unpack Target 8/1 -> Target 8/1
  CAN Unpack Target 2/1 -> Target 2/1
  CAN Unpack Target 1/1 -> Target 1/1
  CAN Unpack Target 4/1 -> Target 4/1
  CAN Unpack Target 5/1 -> Target 5/1
  CAN Unpack Target 7/1 -> Target 7/1
  CAN Unpack Target 6/1 -> Target 6/1
  CAN Unpack Target 0/1 -> Target 0/1
  CAN Unpack Target 9/1 -> Target 9/1

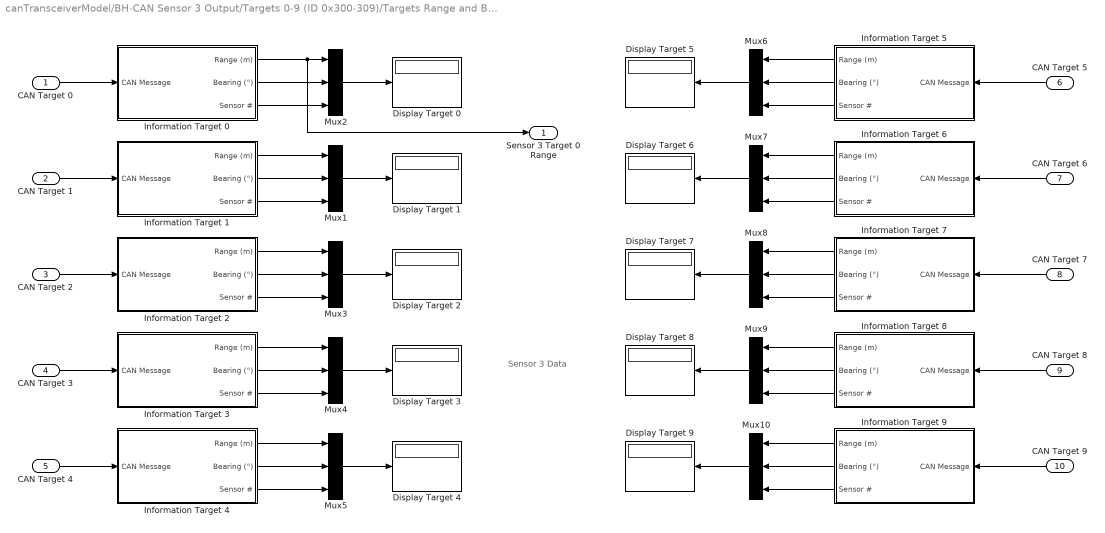
== system canTransceiverModel/BH-CAN Sensor 3 Output/Targets 0-9 (ID 0x300-309)/Targets Range and Bearing Information ==
  note: Sensor 3
      | Data
  CAN Target 0 : Inport
  CAN Target 1 : Inport  Port=2
  CAN Target 2 : Inport  Port=3
  CAN Target 3 : Inport  Port=4
  CAN Target 4 : Inport  Port=5
  CAN Target 5 : Inport  Port=6
  CAN Target 6 : Inport  Port=7
  CAN Target 7 : Inport  Port=8
  CAN Target 8 : Inport  Port=9
  CAN Target 9 : Inport  Port=10
  Display Target {0..9} (10 alike) : Display
  Information Target 0 : Subsystem
  Information Target 1 : Subsystem
  Information Target 2 : Subsystem
  Information Target 3 : Subsystem
  Information Target 4 : Subsystem
  Information Target 5 : Subsystem
  Information Target 6 : Subsystem
  Information Target 7 : Subsystem
  Information Target 8 : Subsystem
  Information Target 9 : Subsystem
  Mux{1..10} (10 alike) : Mux  Inputs=3
  Sensor 3 Target 0 Range : Outport
  wires:
  Information Target 0/2(Bearing (°)) -> Mux2/2
  CAN Target 0/1 -> Information Target 0/1(CAN Message)
  Mux2/1 -> Display Target 0/1
  Information Target 0/3(Sensor #) -> Mux2/3
  CAN Target 1/1 -> Information Target 1/1(CAN Message)
  Information Target 1/3(Sensor #) -> Mux1/3
  Mux1/1 -> Display Target 1/1
  Information Target 1/2(Bearing (°)) -> Mux1/2
  CAN Target 2/1 -> Information Target 2/1(CAN Message)
  Information Target 2/3(Sensor #) -> Mux3/3
  Mux3/1 -> Display Target 2/1
  Information Target 2/2(Bearing (°)) -> Mux3/2
  CAN Target 3/1 -> Information Target 3/1(CAN Message)
  Information Target 3/1(Range (m)) -> Mux4/1
  Information Target 3/3(Sensor #) -> Mux4/3
  Mux4/1 -> Display Target 3/1
  Information Target 3/2(Bearing (°)) -> Mux4/2
  CAN Target 4/1 -> Information Target 4/1(CAN Message)
  Information Target 4/1(Range (m)) -> Mux5/1
  Information Target 4/3(Sensor #) -> Mux5/3
  Mux5/1 -> Display Target 4/1
  Information Target 4/2(Bearing (°)) -> Mux5/2
  CAN Target 5/1 -> Information Target 5/1(CAN Message)
  Information Target 5/1(Range (m)) -> Mux6/1
  Information Target 5/3(Sensor #) -> Mux6/3
  Mux6/1 -> Display Target 5/1
  Information Target 5/2(Bearing (°)) -> Mux6/2
  Information Target 6/2(Bearing (°)) -> Mux7/2
  Mux7/1 -> Display Target 6/1
  Information Target 6/3(Sensor #) -> Mux7/3
  CAN Target 6/1 -> Information Target 6/1(CAN Message)
  Information Target 6/1(Range (m)) -> Mux7/1
  Information Target 7/2(Bearing (°)) -> Mux8/2
  Mux8/1 -> Display Target 7/1
  Information Target 7/3(Sensor #) -> Mux8/3
  CAN Target 7/1 -> Information Target 7/1(CAN Message)
  Information Target 7/1(Range (m)) -> Mux8/1
  Information Target 8/2(Bearing (°)) -> Mux9/2
  Mux9/1 -> Display Target 8/1
  Information Target 8/3(Sensor #) -> Mux9/3
  CAN Target 8/1 -> Information Target 8/1(CAN Message)
  Information Target 8/1(Range (m)) -> Mux9/1
  Information Target 9/2(Bearing (°)) -> Mux10/2
  Mux10/1 -> Display Target 9/1
  Information Target 9/3(Sensor #) -> Mux10/3
  CAN Target 9/1 -> Information Target 9/1(CAN Message)
  Information Target 9/1(Range (m)) -> Mux10/1
  Information Target 0/1(Range (m)) -> Sensor 3 Target 0 Range/1, Mux2/1
  Information Target 2/1(Range (m)) -> Mux3/1
  Information Target 1/1(Range (m)) -> Mux1/1
